simulink library "DoorHndReq"  (R2022a)
settings: Solver=VariableStepAuto  StartTime=0.0  StopTime=10.0  RelTol=1e-3
settings Model: Creator=DELL  LastModifiedBy=liyun

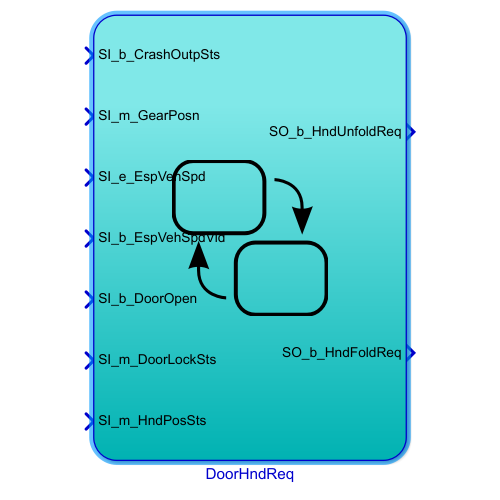
[thumbnail: Simulink's stored preview of the top-level diagram]
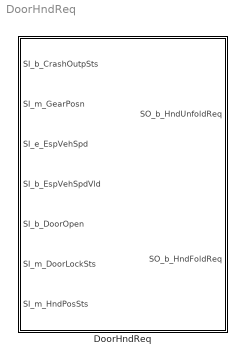
== system DoorHndReq ==
  DoorHndReq : Stateflow chart  TreatAsAtomicUnit=on

== stateflow chart DoorHndReq/DoorHndReq ==
  state AntiPlay [parallel] [commented out]
    state Count [commented out]
      (default) -> (junction 654) [commented out]
      Count -> (junction 654) [commented out]
      (junction 654) -> (junction 655) [commented out] : [hasChangedTo(SI_m_HndPosSts, Hnd_Fold) || ...
          | hasChangedTo(SI_m_HndPosSts, Hnd_Unfold)]
      (junction 654) -> (junction 656) [commented out]
      (junction 655) -> (junction 662) [commented out] : {SL_e_antiPlayCount++;}
      (junction 662) -> (junction 656) [commented out]
      (junction 656) -> (junction 658) [commented out]
    state TrigAndClean [commented out]
      en:
      SL_b_antiPlayFlg = 1;
      SL_e_antiPlayCount = 0;
    state Clean [commented out]
      en:
      SL_e_antiPlayCount = 0;
    (default) -> Count [commented out]
    Count -> TrigAndClean [commented out] : [before(3000, tick) &&...
        | SL_e_antiPlayCount >= 10]
    TrigAndClean -> Count [commented out] : [after(18000, tick)]
        | {SL_b_antiPlayFlg = 0;}
    Count -> Clean [commented out] : [after(3000, tick)]
    Clean -> Count [commented out]
  state Unfold [parallel]
    settings: executionOrder=1
    state Idle
      SO_b_HndUnfoldReq = 0;
    state NormalUnfoldReq
      en:
      SO_b_HndUnfoldReq = 1;
      on at(5, tick):
      SO_b_HndUnfoldReq = 0;
    state CrashUnfoldReq
      en:
      SO_b_HndUnfoldReq = 1;
    (default) -> Unfold.Idle
    Unfold.Idle -> NormalUnfoldReq [order 1] : [SI_e_EspVehSpd < 15 && ...
        | (SI_b_DoorOpen == 1 || SI_m_DoorLockSts == Door_Unlock) && ...
        | SI_m_HndPosSts != Hnd_Unfold]
    NormalUnfoldReq -> Unfold.Idle : [SI_e_EspVehSpd >= 15 || ...
        | (SI_b_DoorOpen == 0 && SI_m_DoorLockSts != Door_Unlock) || ...
        | SI_m_HndPosSts == Hnd_Unfold]
    Unfold.Idle -> CrashUnfoldReq [order 2] : [hasChangedTo(SI_b_CrashOutpSts, 1) && ...
        | SI_m_HndPosSts != Hnd_Unfold]
    CrashUnfoldReq -> Unfold.Idle : after(5, tick)
  state Fold [parallel]
    settings: executionOrder=2
    state Idle
      SO_b_HndFoldReq = 0;
    state FoldReq
      en:
      SO_b_HndFoldReq = 1;
      on at(5, tick):
      SO_b_HndFoldReq = 0;
    (default) -> Fold.Idle
    Fold.Idle -> FoldReq : [SI_m_DoorLockSts == Door_Lock && ...
        | SI_m_HndPosSts != Hnd_Fold]
    FoldReq -> Fold.Idle : [SI_m_DoorLockSts != Door_Lock || ...
        | SI_m_HndPosSts == Hnd_Fold]
  data: SI_b_CrashOutpSts input boolean; SI_m_GearPosn input Enum: Gear_Posn_E; SI_e_EspVehSpd input uint8; SI_b_EspVehSpdVld input boolean; SI_b_DoorOpen input boolean =0; SI_m_DoorLockSts input Enum: Door_Sts_E; SO_b_HndUnfoldReq output boolean; SL_e_antiPlayCount local uint8 =0; SI_m_HndPosSts input Enum: HndPos_Sts_E; SO_b_HndFoldReq output boolean; SL_b_antiPlayFlg local uint8 =0
